simulink model "stateflow"  (R2024a)
settings: Solver=FixedStepDiscrete  StartTime=0.0  StopTime=60.0  FixedStep=0.1  RelTol=1e-3  EnableMultiTasking=on
settings Model: Creator=sn07590  LastModifiedBy=sn07590
settings SolverCC: AlgebraicLoopSolver=TrustRegion  AutoInsertRateTranBlk=on
settings OptimizationCC: LifeSpan=inf
settings DebuggingCC: UnconnectedInputMsg=warning  UnconnectedOutputMsg=warning  UnconnectedLineMsg=warning  SFUnexpectedBacktrackingDiag=warning  SFNoUnconditionalDefaultTransitionDiag=warning  SFExecutionAtInitializationDiag=none  ArithmeticOperatorsInVariantConditions=warning
settings ModelReferenceCC: EnableRefExpFcnMdlSchedulingChecks=on
settings SFSimCC: SimUseLocalCustomCode=off  CustomCodeUndefinedFunction=UseInterfaceOnly
settings RTWCC: RTWUseLocalCustomCode=off  GPUComputeCapability=3.5  DLArmComputeVersion=19.05
settings CodeAppCC: StateflowObjectComments=on
settings GRTTargetCC: TargetLangStandard=C89/C90 (ANSI)
settings ConfigComp: CovMetricSettings=dw  CovSaveCumulativeToWorkspaceVar=on  CovSaveSingleToWorkspaceVar=on  CovExternalEMLEnable=off

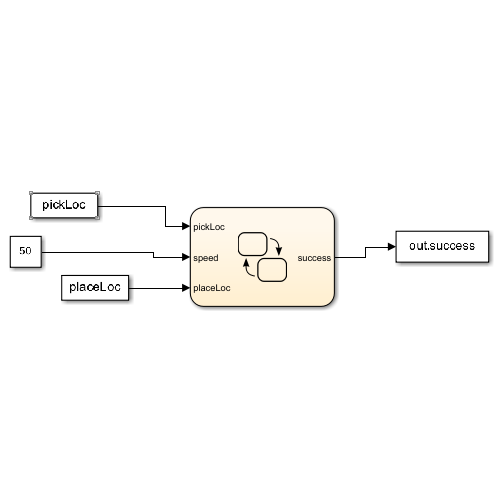
[thumbnail: Simulink's stored preview of the top-level diagram]
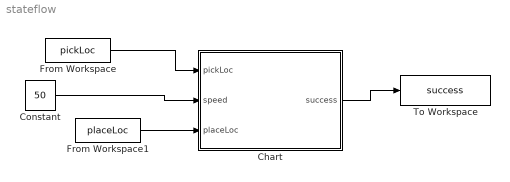
== system stateflow ==
  Chart : Stateflow chart  TreatAsAtomicUnit=on
  Constant : Constant  Value=50
  From Workspace : FromWorkspace  VariableName=pickLoc
  From Workspace1 : FromWorkspace  VariableName=placeLoc
  To Workspace : ToWorkspace  VariableName=success  SaveFormat=Timeseries  SampleTime=-1
  wires:
  From Workspace/1 -> Chart/1(pickLoc)
  From Workspace1/1 -> Chart/3(placeLoc)
  Constant/1 -> Chart/2(speed)
  Chart/1(success) -> To Workspace/1

== stateflow chart stateflow/Chart ==
  state IDLE
    entry:
    utils.initArb()
    success = utils.setPosition([0.5676  -0.7721  0.8641  0.5931  0], speed);
  state Pick % Parent State
    entry:
    state Pregrasp
      entry:
      pose = utils.preGraspPose(pickLoc);
      q = utils.findOptimalSolution(pose(1), pose(2), pose(3), pose(4));
      success = utils.setPosition(q, speed);
    state GraspPose % Child State
      entry:
      q = utils.findOptimalSolution(pose(1), pose(2), pose(3)-5, pose(4));
      success = utils.setPosition(q, speed);
    state PickObject % Child State
      entry:
      success = utils.gripObject(2.6);
    (default) -> Pregrasp
    Pregrasp -> GraspPose % Child State : after(5, sec)[success == 0]
    GraspPose % Child State -> PickObject % Child State : after(5, sec)[success == 0]
  state Place
    state GoToLoc
      entry:
      pose = utils.preGraspPose(placeLoc)
      q = utils.findOptimalSolution(pose(1), pose(2), pose(3)-5, pose(4))
      success = utils.setPosition(q, speed);
    state PlaceObject % Child State
      entry:
      success = utils.gripObject(3.8);
    state PostPlace
      entry:
      pose = utils.preGraspPose(pickLoc);
      q = utils.findOptimalSolution(pose(1), pose(2), pose(3)+10, pose(4));
      success = utils.setPosition(q, speed);
    (default) -> GoToLoc
    GoToLoc -> PlaceObject % Child State : [success == 0]
    PlaceObject % Child State -> PostPlace : [success == 0]
  PostPlace -> IDLE : [success == 0]
  (default) -> Pick % Parent State
  PickObject % Child State -> Place : [success == 0]
  data: pickLoc input size=3; speed input size=1; success output; pose local; q local; placeLoc input size=3
